simulink model "MIT_normalaized"  (R2022b)
settings: Solver=VariableStepAuto  StartTime=0.0  StopTime=6000  RelTol=1e-5
values from neighbouring files (symbols this model uses):
  den_real = [1, (tau1 + tau2 + R2) / (tau1*tau2), 1/ (tau1*tau2)]    [SIMULATION_CODE.m]
  num_real = [R2/(tau1*tau2)]    [SIMULATION_CODE.m]
undefined symbols (not defined in the file or in its folder): den_des, num_des
libraries: dspsrcs4 x1
settings Model: Creator=mahdi  LastModifiedBy=user
settings DebuggingCC: UnconnectedInputMsg=warning  UnconnectedOutputMsg=warning  UnconnectedLineMsg=warning
settings ModelReferenceCC: EnableRefExpFcnMdlSchedulingChecks=on
settings RTWCC: DLArmComputeVersion=19.05

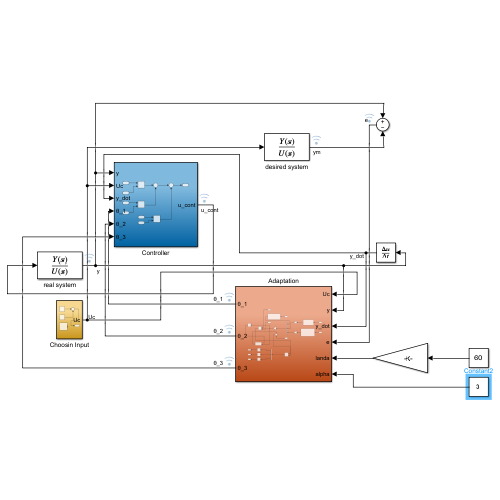
[thumbnail: Simulink's stored preview of the top-level diagram]
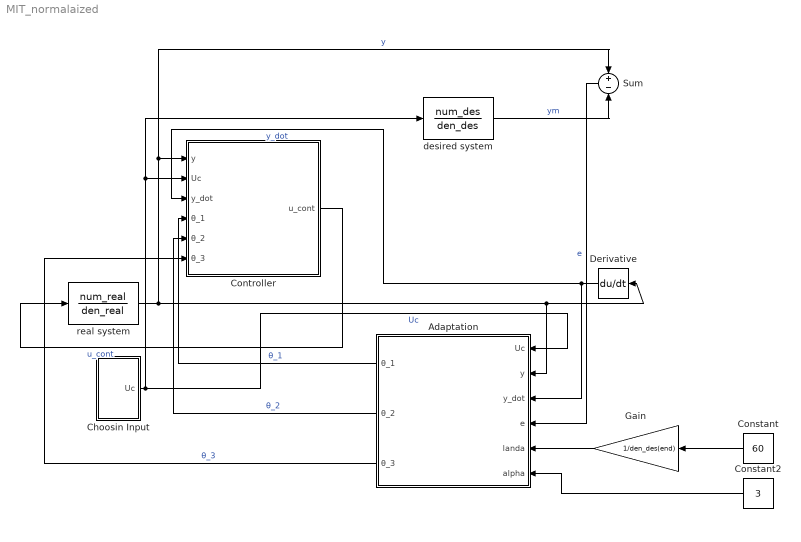
== system MIT_normalaized ==
  Adaptation : Subsystem
  Choosin Input : Subsystem
  Constant : Constant  Value=60
  Constant2 : Constant  Value=3
  Controller : Subsystem
  Derivative : Derivative
  Gain : Gain  Gain=1/den_des(end)
  Sum : Sum  Inputs=+|-
  desired system : TransferFcn  Numerator=num_des  Denominator=den_des
  real system : TransferFcn  Numerator=num_real  Denominator=den_real
  wires:
  Constant/1 -> Gain/1
  Sum/1 -> Adaptation/4(e)  "e"
  Gain/1 -> Adaptation/5(landa)
  real system/1 -> Derivative/1, Adaptation/2(y), Sum/1, Controller/1(y)  "y"
  Choosin Input/1(Uc) -> desired system/1, Controller/2(Uc), Adaptation/1(Uc)  "Uc"
  desired system/1 -> Sum/2  "ym"
  Adaptation/2(θ_2) -> Controller/5(θ_2)  "θ_2"
  Derivative/1 -> Adaptation/3(y_dot), Controller/3(y_dot)  "y_dot"
  Controller/1(u_cont) -> real system/1  "u_cont"
  Adaptation/3(θ_3) -> Controller/6(θ_3)  "θ_3"
  Adaptation/1(θ_1) -> Controller/4(θ_1)  "θ_1"
  Constant2/1 -> Adaptation/6(alpha)

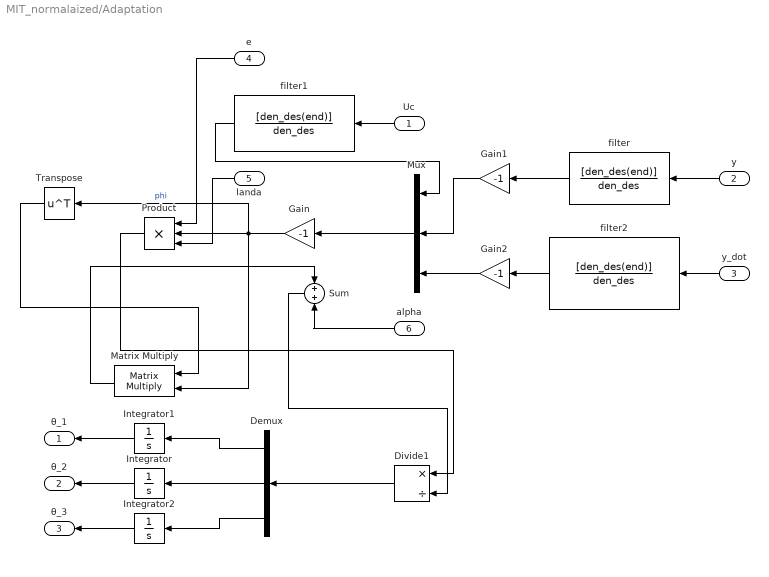
== system MIT_normalaized/Adaptation ==
  Uc : Inport
  y : Inport  Port=2
  y_dot : Inport  Port=3
  e : Inport  Port=4
  landa : Inport  Port=5
  alpha : Inport  Port=6
  Demux : Demux  Outputs=3
  Divide1 : Product  Inputs=*/
  Gain : Gain  Gain=-1
  Gain1 : Gain  Gain=-1
  Gain2 : Gain  Gain=-1
  Integrator : Integrator
  Integrator1 : Integrator
  Integrator2 : Integrator
  Matrix Multiply : Product  Multiplication=Matrix(*)
  Mux : Mux  Inputs=3
  Product : Product  Inputs=3
  Sum : Sum  Inputs=+|+
  Transpose : Math  Operator=transpose
  filter : TransferFcn  Numerator=[den_des(end)]  Denominator=den_des
  filter1 : TransferFcn  Numerator=[den_des(end)]  Denominator=den_des
  filter2 : TransferFcn  Numerator=[den_des(end)]  Denominator=den_des
  θ_1 : Outport
  θ_2 : Outport  Port=2
  θ_3 : Outport  Port=3
  wires:
  e/1 -> Product/1
  Transpose/1 -> Matrix Multiply/1
  Integrator2/1 -> θ_3/1
  landa/1 -> Product/3
  Integrator/1 -> θ_2/1
  y/1 -> filter/1
  Gain1/1 -> Mux/2
  Demux/2 -> Integrator/1
  Integrator1/1 -> θ_1/1
  alpha/1 -> Sum/2
  Matrix Multiply/1 -> Sum/1
  filter1/1 -> Mux/1
  Product/1 -> Divide1/1
  y_dot/1 -> filter2/1
  Demux/3 -> Integrator2/1
  Gain/1 -> Transpose/1, Product/2, Matrix Multiply/2  "phi"
  Sum/1 -> Divide1/2
  Uc/1 -> filter1/1
  Demux/1 -> Integrator1/1
  filter/1 -> Gain1/1
  Mux/1 -> Gain/1
  Divide1/1 -> Demux/1
  filter2/1 -> Gain2/1
  Gain2/1 -> Mux/3

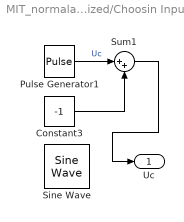
== system MIT_normalaized/Choosin Input ==
  Constant3 : Constant  Value=-1
  Pulse Generator1 : DiscretePulseGenerator  PulseType=Time based  Amplitude=2  Period=3000  PulseWidth=50
  Sine Wave : dspsrcs4/Sine Wave  Amplitude=1  Frequency=0.02  Phase=0  SampleMode=Continuous  OutComplex=Real  CompMethod=Trigonometric fcn  TableSize=Speed  SampleTime=0  SamplesPerFrame=1  ResetState=Restart at time zero  OutputFrames=off  dataType=double  wordLen=16  udDataType=sfix(16)  fracBitsMode=Best precision  numFracBits=15  OutDataTypeStr=double  LastOutDataTypeStr=double
  Sum1 : Sum  Inputs=|++
  Uc : Outport
  wires:
  Constant3/1 -> Sum1/2
  Pulse Generator1/1 -> Sum1/1  "Uc"
  Sum1/1 -> Uc/1

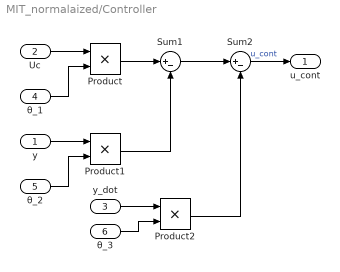
== system MIT_normalaized/Controller ==
  y : Inport
  Uc : Inport  Port=2
  y_dot : Inport  Port=3
  θ_1 : Inport  Port=4
  θ_2 : Inport  Port=5
  θ_3 : Inport  Port=6
  Product : Product
  Product1 : Product
  Product2 : Product
  Sum1 : Sum  Inputs=|+-
  Sum2 : Sum  Inputs=|+-
  u_cont : Outport
  wires:
  θ_3/1 -> Product2/2
  y_dot/1 -> Product2/1
  y/1 -> Product1/1
  Product/1 -> Sum1/1
  θ_2/1 -> Product1/2
  θ_1/1 -> Product/2
  Uc/1 -> Product/1
  Product1/1 -> Sum1/2
  Sum1/1 -> Sum2/1
  Product2/1 -> Sum2/2
  Sum2/1 -> u_cont/1  "u_cont"
